simulink model "B3_fcn"  (R2020b)
settings: Solver=ode45  StartTime=0.0  StopTime=10.0  MaxStep=0.01  RelTol=1e-3  EnableMultiTasking=on
model workspace (MAT data in the model file):
  k = 1
values from neighbouring files (symbols this model uses):
  c = 3    [B2_create_variables.m]    (also in B2_create_variablesA.m = 2)
  m = 1    [B2_create_variables.m]    (also in B2_create_variablesA.m)
settings Model: Creator=Reichl  LastModifiedBy=jakob
settings DataIOCC: LimitDataPoints=on  SaveFormat=Array  SignalLoggingSaveFormat=ModelDataLogs  ReturnWorkspaceOutputs=off
settings OptimizationCC: ExpressionDepthLimit=2147483647  LifeSpan=inf
settings DebuggingCC: UnderspecifiedInitializationDetection=Classic  MergeDetectMultiDrivingBlocksExec=none  SolverPrmCheckMsg=warning  FcnCallInpInsideContextMsg=warning  StateNameClashWarn=warning  SFUnexpectedBacktrackingDiag=warning  SFNoUnconditionalDefaultTransitionDiag=warning  SFExecutionAtInitializationDiag=none  ArithmeticOperatorsInVariantConditions=warning
settings HardwareCC: ProdBitPerPointer=32  ProdBitPerSizeT=32  ProdBitPerPtrDiffT=32  ProdLargestAtomicFloat=None  ProdIntDivRoundTo=Undefined  ProdEndianess=Unspecified  ProdWordSize=32  ProdHWDeviceType=32-bit Generic
settings ModelReferenceCC: PropagateSignalLabelsOutOfModel=off
settings SFSimCC: SimUseLocalCustomCode=off  CustomCodeUndefinedFunction=UseInterfaceOnly
settings RTWCC: RTWUseLocalCustomCode=off
settings CodeAppCC: StateflowObjectComments=on
settings GRTTargetCC: TargetLangStandard=C89/C90 (ANSI)  CombineOutputUpdateFcns=off  GRTInterface=on
settings ConfigComp: CovMetricSettings=dw  CovSaveCumulativeToWorkspaceVar=on  CovSaveSingleToWorkspaceVar=on  CovExternalEMLEnable=off  CovSFcnEnable=off

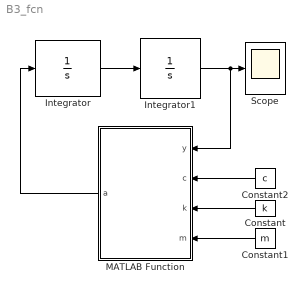
== system B3_fcn ==
  Constant : Constant  Value=k
  Constant1 : Constant  Value=m
  Constant2 : Constant  Value=c
  Integrator : Integrator
  Integrator1 : Integrator  InitialCondition=3
  MATLAB Function : MATLAB Function  TreatAsAtomicUnit=on
  Scope : Scope
  wires:
  Integrator/1 -> Integrator1/1
  Integrator1/1 -> MATLAB Function/1(y), Scope/1
  MATLAB Function/1(a) -> Integrator/1
  Constant2/1 -> MATLAB Function/2(c)
  Constant/1 -> MATLAB Function/3(k)
  Constant1/1 -> MATLAB Function/4(m)

== matlab function B3_fcn/MATLAB Function ==
  data: y input; a output; c input; k input; m input
function a = fcn(y,c,k,m)
% y = u; Defaultverhalten
a = -k/m*y-c/m*y^3;
